simulink model "eml_fire"  (Simulink 7.6)
settings: Solver=FixedStepDiscrete  StartTime=0.0  StopTime=inf  RelTol=1e-3
PreLoadFcn:
  | %load mtlb;
  | 
  | Fs = 8000;
libraries: simulink x1
CloseFcn:
  | rtwprivate ssgencode ModelCloseRequest eml_fire
settings Model: Creator=The MathWorks Inc.  CovMetricSettings=dmw  ExtModeAutoUpdateStatusClock=off
settings DataIOCC: SaveOutput=off  SaveTime=off  SignalLoggingName=logsOut
settings OptimizationCC: InlineInvariantSignals=on  InitFltsAndDblsToZero=on
settings DebuggingCC: SaveWithParameterizedLinksMsg=none  CheckExecutionContextPreStartOutputMsg=on  CheckExecutionContextRuntimeOutputMsg=on  SignalResolutionControl=TryResolveAllWithWarning  SolverPrmCheckMsg=none  MultiTaskDSMMsg=warning  MultiTaskCondExecSysMsg=none  StrictBusMsg=None
settings HardwareCC: TargetUnknown=on
settings SFSimCC: SFSimEcho=off  SimParseCustomCode=off
settings RTWCC: GenerateReport=on  LaunchReport=on  IncludeERTFirstTime=on
settings CodeAppCC: MangleLength=5
settings GRTTargetCC: TargetFcnLib=ansi_tfl_tmw.mat

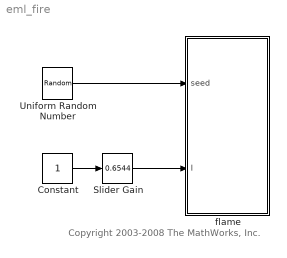
== system eml_fire ==
  note: Copyright 2003-2008 The MathWorks, Inc.
  Constant : Constant
  Slider Gain : simulink/Math Operations/Slider Gain  SystemSampleTime=-1  low=0  gain=0.6544  high=1
  Uniform Random Number : UniformRandomNumber  Minimum=0  Seed=floor(rand(1,256) * 4560458)  SampleTime=0
  flame : Stateflow chart  TreatAsAtomicUnit=on
  wires:
  Constant/1 -> Slider Gain/1
  Slider Gain/1 -> flame/2(I)
  Uniform Random Number/1 -> flame/1(seed)

== matlab function flame ==
  data: seed input double size=1 256; I input double
function flame(seed, I)

persistent p;
if isempty(p)
    p = zeros(64,256,'uint8');
end

WIDTH   = length(seed);
HEIGHT  = size(p,1);
nColors = 256;

nRandTemp = seed;
nRandTemp = abs(nRandTemp) * 2;
nRandTemp = min(nRandTemp,1);

generator = nRandTemp * nColors * I;

for y = 1 : 2 : (HEIGHT-4)
    for x = 1 : WIDTH
        
        yb = y+2;
        xb1 = x-1;
        xb2 = x+1;
        
        if xb1 < 1
            xb1 = WIDTH;
            yb = yb + 1;
        end
        if xb2 > WIDTH
            xb2 = 1;
            yb = yb - 1;
        end
        
        if yb > HEIGHT
            yb = 1;
        end
        
        top    = double(p(yb,x)) + double(p(yb,xb1)) + double(p(yb,xb2));
        bottom = double(p(y+4,x));
        
        c1 = floor((top + bottom) * 0.25);
        
        if c1 > 1
            c1 = c1 - 1;
        end
        
        c2 = floor((c1+bottom) * 0.5);
        
        p(y+2,x)   = uint8(c1);
        p(y+3,x)   = uint8(c2);
        
    end
end

for y = HEIGHT-3 : 2 : HEIGHT
    for x = 1 : WIDTH
        
        yb = y;
        
        if y<HEIGHT-2
            yb = yb + 2;
            xb1 = x - 1;
            if xb1 < 1
                xb1 = WIDTH;
                yb = yb + 1;
            end
            xb2 = x + 1;
            if xb2 > WIDTH
                xb2 = 1;
                yb = yb + 1;
            end
            top = double(p(yb,xb1)) + double(p(yb,x)) + double(p(yb,xb2));
        else
            top = generator(x);
            if x == WIDTH
                top = top + generator(1);
            else
                top = top + generator(x+1);
            end
            
            if x == 1
                top = top + generator(WIDTH);
            else
                top = top + generator(x - 1);
            end
        end
        
        bottom = generator(x);
        
        c1 = floor((top + bottom) * 0.25);
        if c1 > 1
            c1 = c1 - 1;
        end
        
        c2 = floor((c1+bottom) * 0.5);
        
        if yb<HEIGHT
            p(yb,   x) = uint8(c1);
            p(yb+1, x) = uint8(c2);
        end
    end
end
eml.extrinsic('fire_show');
fire_show(p);
